simulink model "MagLevLinearModel"  (R2015b)
settings: Solver=VariableStepAuto  StartTime=0.0  StopTime=10.0  RelTol=1e-3
values from neighbouring files (symbols this model uses):
  delta_V = V-v_o    [LinearizeModelSimulation.m]
  i_o = 1.0005    [LinearizeModelSimulation.m]
  Km = 6.5308*10^-5    (= 6.5308e-05)    [LinearizeModelSimulation.m]
  L = 0.4125    [LinearizeModelSimulation.m]
  Mb = 0.068    [LinearizeModelSimulation.m]
  Rc = 10    [LinearizeModelSimulation.m]
  Rs = 1    [LinearizeModelSimulation.m]
  v_o = 11.0055    [LinearizeModelSimulation.m]
  x_o = 0.007    [LinearizeModelSimulation.m]
settings Model: Creator=Christopher  LastModifiedBy=Christopher
settings ConfigComp: CovModelRefEnable=Off

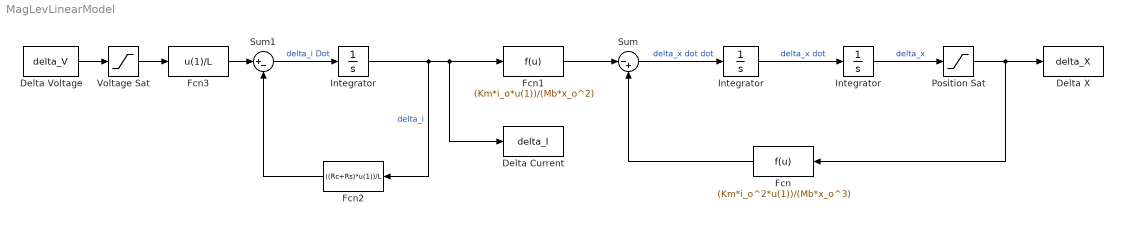
== system MagLevLinearModel ==
  Delta Current : ToWorkspace  VariableName=delta_I  SaveFormat=Structure With Time  SampleTime=-1
  Delta Voltage : Constant  Value=delta_V
  Delta X : ToWorkspace  VariableName=delta_X  SaveFormat=Structure With Time  SampleTime=-1
  Fcn : Fcn  Expr=(Km*i_o^2*u(1))/(Mb*x_o^3)
  Fcn1 : Fcn  Expr=(Km*i_o*u(1))/(Mb*x_o^2)
  Fcn2 : Fcn  Expr=((Rc+Rs)*u(1))/L
  Fcn3 : Fcn  Expr=u(1)/L
  Integrator : Integrator  InitialCondition=0-x_o
  "Integrator " : Integrator  InitialCondition=0-i_o
  "Integrator " : Integrator  InitialCondition=0.014-x_o
  Position Sat : Saturate  UpperLimit=0.014-x_o  LowerLimit=0.00001-x_o
  Sum : Sum  Inputs=|-+
  Sum1 : Sum  Inputs=|+-
  Voltage Sat : Saturate  UpperLimit=24-v_o  LowerLimit=-24-v_o
  wires:
  Sum/1 -> Integrator/1  "delta_x dot dot"
  Integrator/1 -> "Integrator "/1  "delta_x dot"
  "Integrator "/1 -> Position Sat/1  "delta_x"
  Fcn/1 -> Sum/2
  Fcn1/1 -> Sum/1
  Fcn3/1 -> Sum1/1
  Sum1/1 -> "Integrator "/1  "delta_i Dot"
  "Integrator "/1 -> Delta Current/1, Fcn1/1, Fcn2/1  "delta_i"
  Fcn2/1 -> Sum1/2
  Position Sat/1 -> Delta X/1, Fcn/1
  Voltage Sat/1 -> Fcn3/1
  Delta Voltage/1 -> Voltage Sat/1
